simulink model "fig4_5_simulink"  (R2021b)
settings: Solver=ode3  StartTime=0.0  StopTime=1000  FixedStep=1e-03  RelTol=1e-3  EnableMultiTasking=on
settings Model: Creator=Nima  LastModifiedBy=One Informatic
settings SolverCC: AlgebraicLoopSolver=TrustRegion
settings DataIOCC: LimitDataPoints=on  SaveFormat=Array  ReturnWorkspaceOutputs=off
settings OptimizationCC: LifeSpan=inf
settings DebuggingCC: SolverPrmCheckMsg=warning  SFUnexpectedBacktrackingDiag=warning  SFNoUnconditionalDefaultTransitionDiag=warning  SFExecutionAtInitializationDiag=none  SFMachineParentedDataDiag=warning  ArithmeticOperatorsInVariantConditions=warning
settings HardwareCC: ProdBitPerPointer=32  ProdBitPerSizeT=32  ProdBitPerPtrDiffT=32  ProdLargestAtomicFloat=None  ProdIntDivRoundTo=Undefined  ProdEndianess=Unspecified  ProdWordSize=32  ProdHWDeviceType=32-bit Generic
settings ModelReferenceCC: PropagateSignalLabelsOutOfModel=off
settings SFSimCC: SimUseLocalCustomCode=off  CustomCodeUndefinedFunction=UseInterfaceOnly
settings RTWCC: RTWUseLocalCustomCode=off
settings CodeAppCC: StateflowObjectComments=on
settings GRTTargetCC: TargetLangStandard=C89/C90 (ANSI)
settings ConfigComp: CovMetricSettings=dw  CovSaveCumulativeToWorkspaceVar=on  CovSaveSingleToWorkspaceVar=on  CovExternalEMLEnable=off  CovSFcnEnable=off

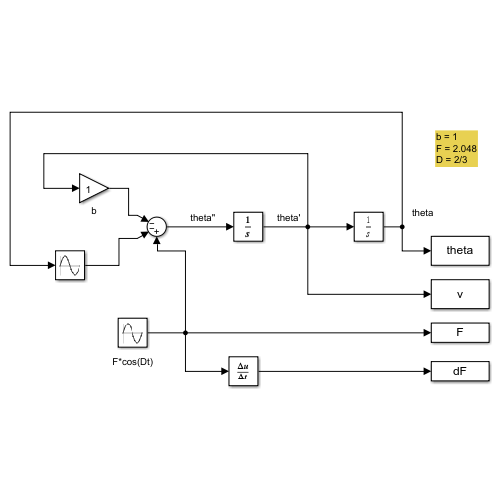
[thumbnail: Simulink's stored preview of the top-level diagram]
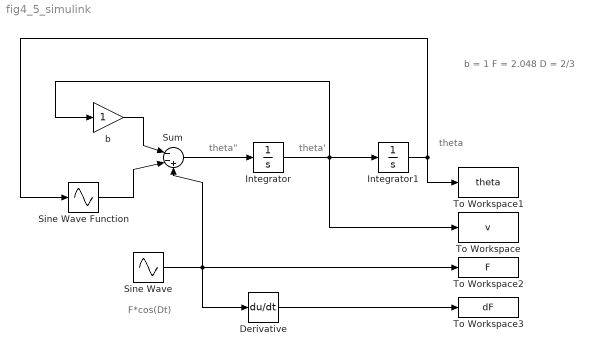
== system fig4_5_simulink ==
  note: b = 1
      | F = 2.048
      | D = 2/3
  note: F*cos(Dt)
  note: theta"
  note: theta'
  note: theta
  Derivative : Derivative
  Integrator : Integrator  InitialCondition=0.01
  Integrator1 : Integrator  InitialCondition=0.01
  Sine Wave : Sin  Amplitude=2.048  Frequency=2/3  SampleTime=0
  Sine Wave Function : Sin  TimeSource=Use external signal  SampleTime=0
  Sum : Sum  Inputs=|--+
  To Workspace : ToWorkspace  VariableName=v  SaveFormat=Timeseries  SampleTime=-1
  To Workspace1 : ToWorkspace  VariableName=theta  SaveFormat=Timeseries  SampleTime=-1
  To Workspace2 : ToWorkspace  VariableName=F  SaveFormat=Timeseries  SampleTime=-1
  To Workspace3 : ToWorkspace  VariableName=dF  SaveFormat=Timeseries  SampleTime=-1
  b : Gain
  wires:
  b/1 -> Sum/1
  Sine Wave Function/1 -> Sum/2
  Sum/1 -> Integrator/1
  Integrator/1 -> b/1, Integrator1/1, To Workspace/1
  Integrator1/1 -> Sine Wave Function/1, To Workspace1/1
  Sine Wave/1 -> Derivative/1, Sum/3, To Workspace2/1
  Derivative/1 -> To Workspace3/1
